simulink model "model"  (R2020b)
settings: Solver=VariableStepAuto  StartTime=0.0  StopTime=100  RelTol=1e-3
undefined symbols (not defined in the file or in its folder): sigbuilder_block
settings Model: PacingRate=1.100000  Creator=Pavan  LastModifiedBy=Pavan

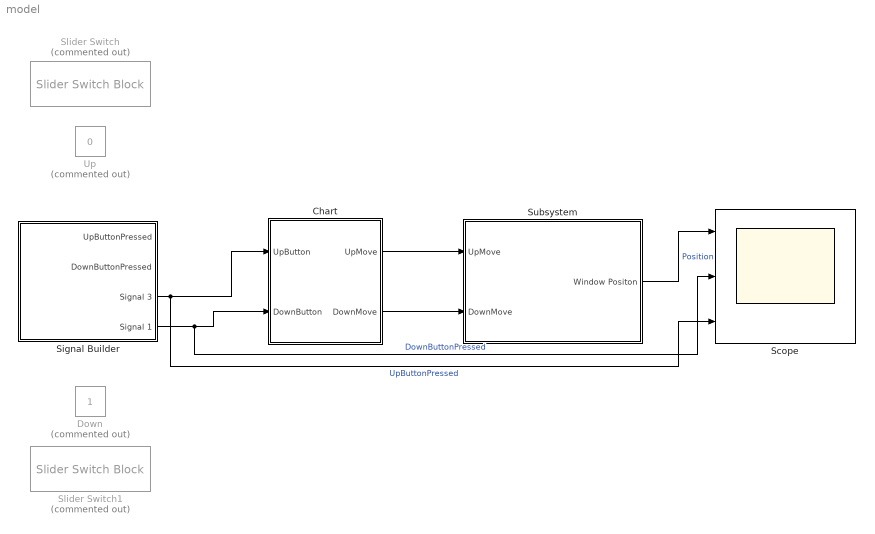
== system model ==
  Chart : Stateflow chart  TreatAsAtomicUnit=on
  Down : Constant  Commented=on
  Scope : Scope  NumInputPorts=3
  Signal Builder : Subsystem  Tag=STV Subsys  LoadFcn=sigbuilder_block('load',[437.6 153 550.4 359.25 ]);  StartFcn=sigbuilder_block('start');  StopFcn=sigbuilder_block('stop');  ClipboardFcn=sigbuilder_block('clipboard');  mask(Sigbuilder block){tuvar=[0:10]}
      mask help: Simulink:masks:SigbuilderBlock_MD
      mask init:
      | if ~strcmp(get_param(bdroot(gcbh),'SimulationStatus'),'stopped') tuvar = sigbuilder_block('maskInit'); end
      settings: CopyFcn=sigbuilder_block('copy');  DeleteFcn=sigbuilder_block('delete');  ModelCloseFcn=sigbuilder_block('modelClose');  PreSaveFcn=sigbuilder_block('preSave');  PauseFcn=sigbuilder_block('pause');  ContinueFcn=sigbuilder_block('continue');  NameChangeFcn=sigbuilder_block('namechange');  OpenFcn=sigbuilder_block('open',[437.6 153 550.4 359.25 ]);  CloseFcn=sigbuilder_block('close');
      mask Display: plot(0, 0, 100, 100,[2, 2, 32, 32, 2], [68, 8, 8, 68, 68],[32, 2], [38, 38], [32, 19, 2],[53, 60, 44], [32, 17, 17, 2],[16, 16, 31, 31]);txt = getActiveGroup(gcbh);text(2, 100, txt,'verticalAlignment', 'top');
  Slider Switch : SliderSwitchBlock  Commented=on
      settings: Values={{'Off', 'On'}, [0 1]}
  Slider Switch1 : SliderSwitchBlock  Commented=on
      settings: Values={{'Off', 'On'}, [0 1]}
  Subsystem : Subsystem
  Up : Constant  Commented=on  Value=0
  wires:
  Chart/1(UpMove) -> Subsystem/1(UpMove)
  Chart/2(DownMove) -> Subsystem/2(DownMove)
  Subsystem/1(Window Positon) -> Scope/1  "Position"
  Signal Builder/3(Signal 3) -> Scope/3, Chart/1(UpButton)  "UpButtonPressed"
  Signal Builder/4(Signal 1) -> Scope/2, Chart/2(DownButton)  "DownButtonPressed"

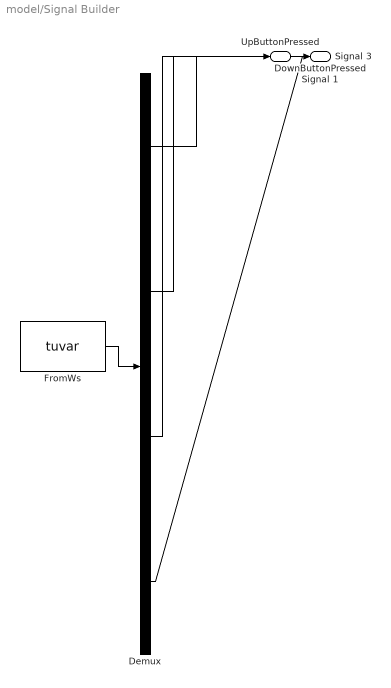
== system model/Signal Builder ==
  Demux : Demux  Tag=STV Demux
      settings: DisplayOption=none
  FromWs : FromWorkspace  Tag=STV FromWs  VariableName=tuvar
      SigBuilderData=|
      | common.afterFinalStr = 'Extrapolate'
      | common.sampleTime = 0
      | dataSet.timeRange = [0 100]
      | dataSet.name = 'Group 1'
      | sbobj.Groups.Name = 'Group 1'
      | sbobj.Groups.Signals(1).Name = 'UpButtonPressed'
      | sbobj.Groups.Signals(1).XData = [0 1 1 5.02 5.02 100]
      | sbobj.Groups.Signals(1).YData = [0 0 1 1 0 0]
      | sbobj.Groups.Signals(2).Name = 'DownButtonPressed'
      | sbobj.Groups.Signals(2).XData = [0 6.02 6.02 100]
      | sbobj.Groups.Signals(2).YData = [0 0 1 1]
      | sbobj.Groups.Signals(3).Name = 'Signal 3'
      | sbobj.Groups.Signals(3).XData = [0 5 5 15 15 20 30 40 40 50 50 70 70 74.8 74.8 95 100]
      | sbobj.Groups.Signals(3).YData = [0 0 1 1 0 0 0 0 1 1 0 0 1 1 0 0 0]
      | sbobj.Groups.Signals(4).Name = 'Signal 1'
      | sbobj.Groups.Signals(4).XData = [0 19.8 19.8 30 30 55 55 60.2 60.2 85 85 100]
      | sbobj.Groups.Signals(4).YData = [0 0 1 1 0 0 1 1 0 0 1 1]
      | sbobj.Groups.TimeRange = [0 100]
  UpButtonPressed : Outport  Tag=STV Outport
  DownButtonPressed : Outport  Tag=STV Outport  Port=2
  Signal 3 : Outport  Tag=STV Outport  Port=3
  Signal 1 : Outport  Tag=STV Outport  Port=4
  wires:
  FromWs/1 -> Demux/1
  Demux/1 -> UpButtonPressed/1
  Demux/2 -> DownButtonPressed/1
  Demux/3 -> Signal 3/1
  Demux/4 -> Signal 1/1

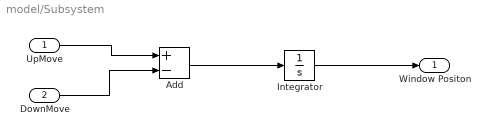
== system model/Subsystem ==
  UpMove : Inport
  DownMove : Inport  Port=2
  Add : Sum  Inputs=+-
  Integrator : Integrator  LimitOutput=on  UpperSaturationLimit=10  LowerSaturationLimit=0
  Window Positon : Outport
  wires:
  UpMove/1 -> Add/1
  Integrator/1 -> Window Positon/1
  DownMove/1 -> Add/2
  Add/1 -> Integrator/1

== stateflow chart model/Chart ==
  state logic
    state switch [parallel]
      en:
      du:
      checkButton()
      settings: executionOrder=1
      state checkButton [function]
        (default) -> (junction 89) : % CheckButton
        (junction 89) -> (junction 90) [order 1] : [UpButton==1&&DownButton==0]
        (junction 89) -> (junction 91) [order 2]
        (junction 90) -> (junction 95) : {send(UP,move);}
        (junction 91) -> (junction 92) [order 1] : [UpButton==0&&DownButton==1]
        (junction 91) -> (junction 93) [order 2] : {send(NEUTRAL,move);}
        (junction 92) -> (junction 94) : {send(DOWN,move);}
        (junction 93) -> (junction 96)
        (junction 94) -> (junction 93)
        (junction 95) -> (junction 94)
    state move [parallel]
      settings: executionOrder=2
      state down
        en:UpMove = 0
        DownMove=1
      state neutral
        en:UpMove = 0
        DownMove=0
      state up
        en: UpMove = 1
        DownMove=0
      down -> up [order 1] : UP
      (default) -> neutral
      neutral -> down [order 2] : DOWN
      neutral -> up [order 1] : UP
      up -> neutral [order 2] : NEUTRAL
      down -> neutral [order 2] : NEUTRAL
      up -> down [order 1] : DOWN
  data: UpMove output; UpButton input; DownMove output; DownButton input
  events: UP local FUNCTION_CALL_EVENT; DOWN local FUNCTION_CALL_EVENT; NEUTRAL local FUNCTION_CALL_EVENT
